simulink model "q_qube2_swingup"  (R2021a)
settings: Solver=ode1  StartTime=0.0  StopTime=10  FixedStep=0.002  RelTol=1e-3  EnableMultiTasking=on
undefined symbols (not defined in the file): a_max, E_r, g, HIL, Jp, k_e, K_unstable, km, l, mp, mr, qc_get_step_size, r, Rm
libraries: quarc_library x3, simulink x1
settings Model: SimulationMode=external  ExtModeTrigDuration=10000  Creator=MLevis  LastModifiedBy=magd4814
settings SolverCC: AlgebraicLoopSolver=TrustRegion  PositivePriorityOrder=on
settings DebuggingCC: UnderspecifiedInitializationDetection=Classic  MergeDetectMultiDrivingBlocksExec=none  SFMachineParentedDataDiag=warning
settings ModelReferenceCC: PropagateSignalLabelsOutOfModel=off
settings SFSimCC: CustomCodeUndefinedFunction=UseInterfaceOnly
settings RTWCC: Description=QUARC Win64 Target Using Toolchain  SystemTargetFile=quarc_win64.tlc  TemplateMakefile=quarc_default_tmf  Toolchain=QUARC win64 | nmake (64-bit Windows)  BuildConfiguration=Faster Runs
settings STFCustomTargetCC: TargetLangStandard=C99 (ISO)  ConcurrentExecutionCompliant=on  SystemTargetFile=quarc_win64.tlc
settings GRTTargetCC: ParMdlRefBuildCompliant=off  CompOptLevelCompliant=off  CombineOutputUpdateFcns=off  MatFileLogging=off  CPPClassGenCompliant=off  GRTInterface=on  ExtMode=on  ExtModeMexFile=quarc_comm

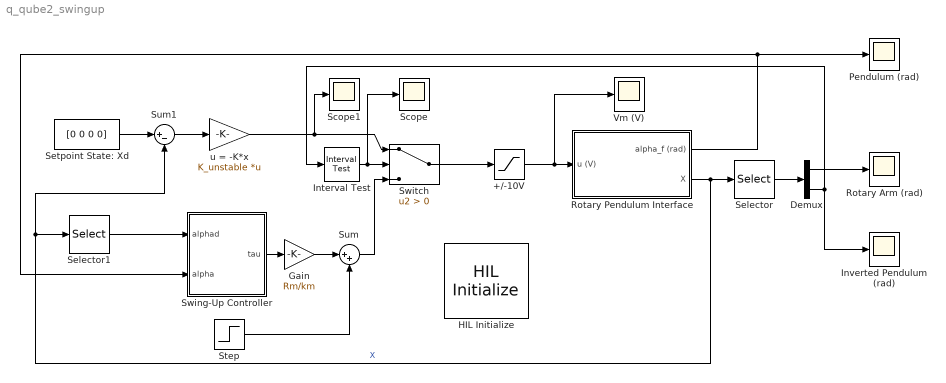
== system q_qube2_swingup ==
  +/-10V : Saturate  UpperLimit=10  LowerLimit=-10
  Demux : Demux  Outputs=2
  Gain : Gain  Gain=Rm/km
  HIL Initialize : quarc_library/Data Acquisition/Generic/Configuration/HIL Initialize  object_name=HIL-1  board_type=qube_servo_usb  board_number=0  board_options=d0=pwm;d1=pwm;led=auto;update_rate=normal;decimation=1  exclusive=off  active=on  hardware_clocks=[0]  clock_modes=[]  initial_clock_frequencies=[]  set_clock_params_at_start=off  set_clock_params_at_switch_in=off  set_clock_frequencies_at_start=off  set_clock_frequencies_at_switch_in=off  analog_input_channels=[]  analog_input_configurations=[]  analog_input_maximums=[]  analog_input_minimums=[]  set_analog_input_params_at_start=off  set_analog_input_params_at_switch_in=off  analog_output_channels=0  analog_output_maximums=10  analog_output_minimums=-10  initial_analog_outputs=[0]  final_analog_outputs=[0]  watchdog_analog_outputs=0  set_analog_output_params_at_start=on  set_analog_output_params_at_switch_in=off  set_analog_outputs_at_start=on  set_analog_outputs_at_switch_in=off  set_analog_outputs_at_terminate=on  set_analog_outputs_at_switch_out=off  set_analog_outputs_on_watchdog=off  digital_input_channels=[]  digital_output_channels=[]  digital_output_configuration=[]  initial_digital_outputs=[]  final_digital_outputs=[]  watchdog_digital_outputs=[]  set_digital_output_params_at_start=off  set_digital_output_params_at_switch_in=off  set_digital_outputs_at_start=off  set_digital_outputs_at_switch_in=off  set_digital_outputs_at_terminate=off  set_digital_outputs_at_switch_out=off  set_digital_outputs_on_watchdog=off  encoder_channels=[0:1]  quadrature=[4]  encoder_filter_frequency=[]  initial_encoder_counts=[0]  set_encoder_params_at_start=on  set_encoder_params_at_switch_in=off  set_encoder_counts_at_start=on  set_encoder_counts_at_switch_in=off  pwm_channels=[]  pwm_modes=[]  pwm_frequency=[]  pwm_configuration=[]  pwm_alignment=[]  pwm_polarity=[]  pwm_leading_deadband=[]  pwm_trailing_deadband=[]  initial_pwm_outputs=[]  final_pwm_outputs=[]  watchdog_pwm_outputs=[]  set_pwm_params_at_start=off  set_pwm_params_at_switch_in=off  set_pwm_outputs_at_start=off  set_pwm_outputs_at_switch_in=off  set_pwm_outputs_at_terminate=off  set_pwm_outputs_at_switch_out=off  set_pwm_outputs_on_watchdog=off  other_output_channels=[]  initial_other_outputs=[]  final_other_outputs=[]  watchdog_other_outputs=[]  set_other_outputs_at_start=off  set_other_outputs_at_switch_in=off  set_other_outputs_at_terminate=off  set_other_outputs_at_switch_out=off  set_other_outputs_on_watchdog=off
  Interval Test : simulink/Logic and Bit Operations/Interval Test  IntervalClosedRight=on  uplimit=0.15*pi  IntervalClosedLeft=on  lowlimit=-0.15*pi  OutDataTypeStr=uint8
  Inverted Pendulum (rad) : Scope
  Pendulum (rad) : Scope
  Rotary Arm (rad) : Scope
  Rotary Pendulum Interface : Subsystem
  Scope : Scope
  Scope1 : Scope
  Selector : Selector  InputPortWidth=4  IndexOptions=Index vector (dialog)  Indices=[1 2]  OutputSizes=1
  Selector1 : Selector  InputPortWidth=4  IndexOptions=Index vector (dialog)  Indices=[4]  OutputSizes=1
  Setpoint State: Xd : Constant  Value=[0 0 0 0]
  Step : Step  Time=0.1  Before=10  After=0  SampleTime=0
  Sum : Sum  Inputs=|++
  Sum1 : Sum  Inputs=|+-
  Swing-Up Controller : Subsystem
  Switch : Switch  Criteria=u2 > Threshold
  Vm (V) : Scope
  u = -K*x : Gain  Gain=K_unstable  Multiplication=Matrix(K*u)
  wires:
  Demux/2 -> Inverted Pendulum (rad)/1, Interval Test/1
  Switch/1 -> +/-10V/1
  Selector/1 -> Demux/1
  +/-10V/1 -> Rotary Pendulum Interface/1(u (V)), Vm (V)/1
  Rotary Pendulum Interface/1(alpha_f (rad)) -> Swing-Up Controller/2(alpha), Pendulum (rad)/1
  Demux/1 -> Rotary Arm (rad)/1
  Interval Test/1 -> Scope/1, Switch/2
  Selector1/1 -> Swing-Up Controller/1(alphad)
  Sum/1 -> Switch/3
  Swing-Up Controller/1(tau) -> Gain/1
  Step/1 -> Sum/2
  Setpoint State: Xd/1 -> Sum1/1
  Sum1/1 -> u = -K*x/1
  Rotary Pendulum Interface/2(X) -> Selector1/1, Sum1/2, Selector/1  "X"
  u = -K*x/1 -> Scope1/1, Switch/1
  Gain/1 -> Sum/1

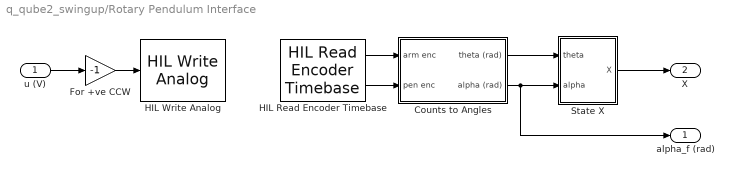
== system q_qube2_swingup/Rotary Pendulum Interface ==
  u (V) : Inport
  Counts to Angles : Subsystem
  For +ve CCW : Gain  Gain=-1
  HIL Read Encoder Timebase : quarc_library/Data Acquisition/Generic/Timebases/HIL Read Encoder Timebase  object_name=HIL-1  clock=0  channels=[0:1]  active=on  vector_output=off  data_type_mode=Inherit via back propagation  data_type=double  overflow_mode=Error on overflow  samples_in_buffer=max(ceil(1/qc_get_step_size), 1)
  HIL Write Analog : quarc_library/Data Acquisition/Generic/Immediate I//O/HIL Write Analog  object_name=HIL-1  channels=0  sample_time=-1  active=on  vector_input=off
  State X : Subsystem
  alpha_f (rad) : Outport  VectorParamsAs1DForOutWhenUnconnected=off
  X : Outport  Port=2  VectorParamsAs1DForOutWhenUnconnected=off
  wires:
  For +ve CCW/1 -> HIL Write Analog/1
  Counts to Angles/2(alpha (rad)) -> alpha_f (rad)/1, State X/2(alpha)
  Counts to Angles/1(theta (rad)) -> State X/1(theta)
  State X/1(X) -> X/1
  u (V)/1 -> For +ve CCW/1
  HIL Read Encoder Timebase/1 -> Counts to Angles/1(arm enc)
  HIL Read Encoder Timebase/2 -> Counts to Angles/2(pen enc)

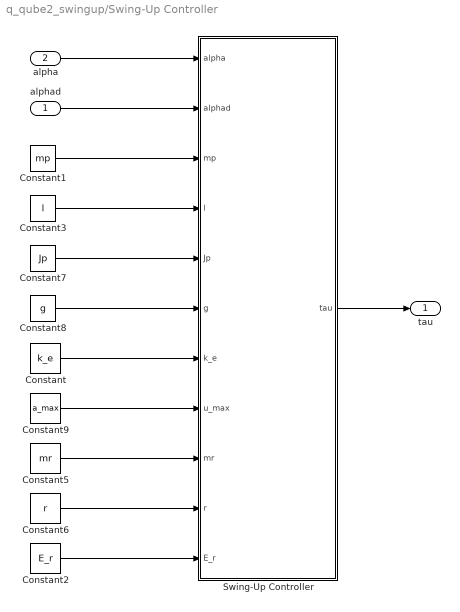
== system q_qube2_swingup/Swing-Up Controller ==
  alphad : Inport
  alpha : Inport  Port=2
  Constant : Constant  Value=k_e
  Constant1 : Constant  Value=mp
  Constant2 : Constant  Value=E_r
  Constant3 : Constant  Value=l
  Constant5 : Constant  Value=mr
  Constant6 : Constant  Value=r
  Constant7 : Constant  Value=Jp
  Constant8 : Constant  Value=g
  Constant9 : Constant  Value=a_max
  Swing-Up Controller : MATLAB Function  TreatAsAtomicUnit=on
  tau : Outport
  wires:
  Constant7/1 -> Swing-Up Controller/5(Jp)
  Constant8/1 -> Swing-Up Controller/6(g)
  Constant1/1 -> Swing-Up Controller/3(mp)
  Constant3/1 -> Swing-Up Controller/4(l)
  Swing-Up Controller/1(tau) -> tau/1
  alphad/1 -> Swing-Up Controller/2(alphad)
  alpha/1 -> Swing-Up Controller/1(alpha)
  Constant/1 -> Swing-Up Controller/7(k_e)
  Constant9/1 -> Swing-Up Controller/8(u_max)
  Constant5/1 -> Swing-Up Controller/9(mr)
  Constant6/1 -> Swing-Up Controller/10(r)
  Constant2/1 -> Swing-Up Controller/11(E_r)

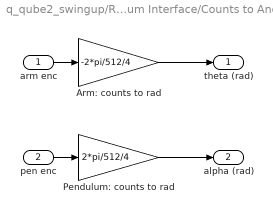
== system q_qube2_swingup/Rotary Pendulum Interface/Counts to Angles ==
  arm enc : Inport
  pen enc : Inport  Port=2
  Arm: counts to rad : Gain  Gain=-2*pi/512/4
  Pendulum: counts to rad : Gain  Gain=2*pi/512/4
  theta (rad) : Outport  VectorParamsAs1DForOutWhenUnconnected=off
  alpha (rad) : Outport  Port=2  VectorParamsAs1DForOutWhenUnconnected=off
  wires:
  pen enc/1 -> Pendulum: counts to rad/1
  arm enc/1 -> Arm: counts to rad/1
  Arm: counts to rad/1 -> theta (rad)/1
  Pendulum: counts to rad/1 -> alpha (rad)/1

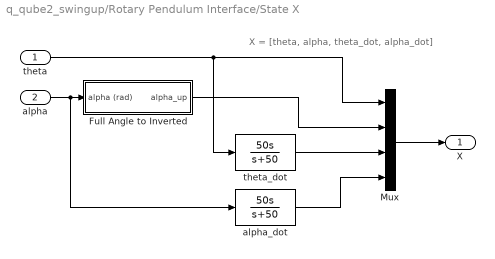
== system q_qube2_swingup/Rotary Pendulum Interface/State X ==
  note: X = [theta, alpha, theta_dot, alpha_dot]
  theta : Inport
  alpha : Inport  Port=2
  Full Angle to Inverted : Subsystem
  Mux : Mux
  alpha_dot : TransferFcn  Numerator=[50 0]  Denominator=[1 50]
  theta_dot : TransferFcn  Numerator=[50 0]  Denominator=[1 50]
  X : Outport  VectorParamsAs1DForOutWhenUnconnected=off
  wires:
  Mux/1 -> X/1
  alpha/1 -> alpha_dot/1, Full Angle to Inverted/1(alpha (rad))
  Full Angle to Inverted/1(alpha_up) -> Mux/2
  theta/1 -> theta_dot/1, Mux/1
  theta_dot/1 -> Mux/3
  alpha_dot/1 -> Mux/4

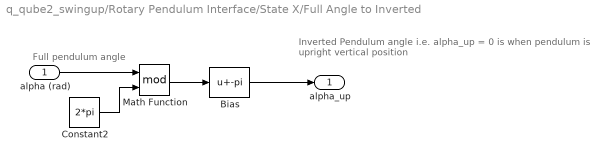
== system q_qube2_swingup/Rotary Pendulum Interface/State X/Full Angle to Inverted ==
  note: Inverted Pendulum angle
      | i.e. alpha_up = 0 is when pendulum is upright vertical position
  note: Full pendulum angle
  alpha (rad) : Inport
  Bias : Bias  Bias=-pi
  Constant2 : Constant  Value=2*pi
  Math Function : Math  Operator=mod  SignedPower=on  SaturateOnIntegerOverflow=on
  alpha_up : Outport  VectorParamsAs1DForOutWhenUnconnected=off
  wires:
  Constant2/1 -> Math Function/2
  alpha (rad)/1 -> Math Function/1
  Bias/1 -> alpha_up/1
  Math Function/1 -> Bias/1

== matlab function q_qube2_swingup/Swing-Up Controller/Swing-Up Controller ==
  data: alpha input; tau output; alphad input; mp input; l input; Jp input; g input; k_e input; u_max input; mr input; r input; E_r input
function tau = fcn(alpha, alphad, mp, l, Jp, g, k_e, u_max, mr, r, E_r)

E = 1/2*Jp*alphad^2 + mp*g*l*(1-cos(alpha));

tau = (mr*r)*u_max*(k_e*(E-E_r)*sign(alphad*cos(alpha)));
